simulink model "district_heating_r02"  (R2018b)
settings: Solver=VariableStepAuto  StartTime=0.0  StopTime=24*3600  RelTol=1e-3
undefined symbols (not defined in the file): CollectorBar, DistributorBar, DPConstant, DPLinear, DPQuadratic, FluidMix, ID, MassFlow, path_carnot, Temperature
libraries: carnot x14, Pipe_BiFlow x2
settings Model: Creator=drhf  LastModifiedBy=drhf
settings SolverCC: AlgebraicLoopSolver=LineSearch

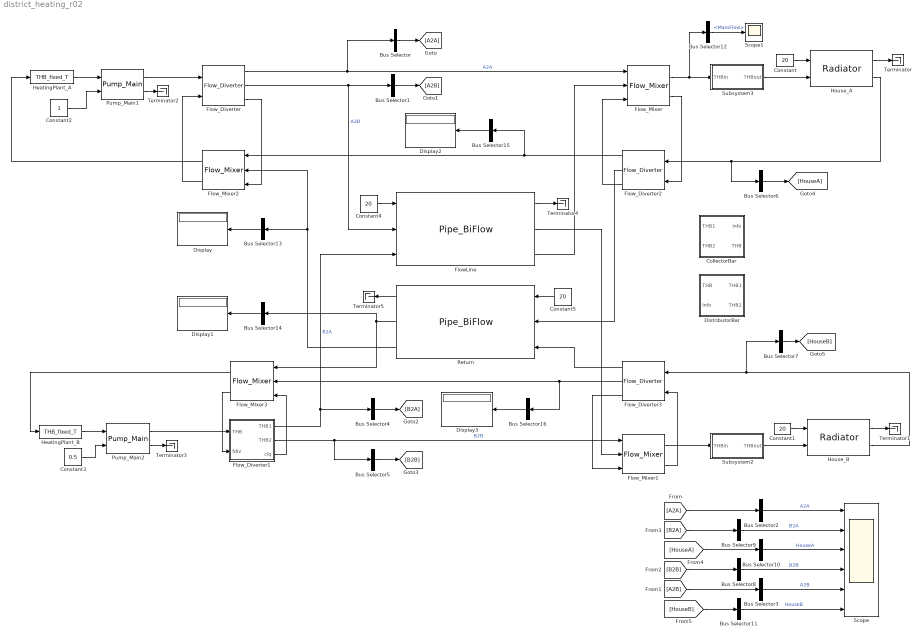
== system district_heating_r02 ==
  Bus Selector{,1,4..7} (6 alike) : BusSelector  OutputSignals=Temperature,MassFlow  OutputAsBus=on
  Bus Selector{2..3,8..11} (6 alike) : BusSelector  OutputSignals=MassFlow  OutputAsBus=on
  Bus Selector12 : BusSelector  OutputSignals=MassFlow
  Bus Selector{13..16} (4 alike) : BusSelector  OutputSignals=DPConstant,DPLinear,DPQuadratic  OutputAsBus=on
  CollectorBar : Subsystem  AncestorBlock=CollectorBar/CollectorBar  mask(Collector bar){}
      mask help: Mixes two massflows. The new temperature is calculated by an energy balance. The "Info" output may be fed back to the corresponding distributor bar.
      mask Help: web(fullfile(path_carnot('help'),'Flow_Mixer.html'),'-helpbrowser')
      mask Display:
      | plot(-50,0, 100,100, ...
      |     [60,60,40,40,60],[10,90,90,10,10], ...
      |     [40,30,30,40],[30,30,20,20], ...
      |     [40,30,30,40],[80,80,70,70], ...
      |     [15,25,15],[30,25,20], ...
      |     [0,25],[25,25], ...
      |     [15,25,15],[80,75,70], ...
      |     [0,25],[75,75])
  Constant{,1,4..5} (4 alike) : Constant  Value=20
  Constant2 : Constant
  Constant3 : Constant  Value=0.5
  Display{,1..3} (4 alike) : Display
  DistributorBar : Subsystem  AncestorBlock=DistributorBar/DistributorBar
      mask Display:
      | plot(0,0,150,100, ...
      |     [60,60,40,40,60],[10,90,90,10,10], ...
      |     [60,70,70,60],[30,30,20,20], ...
      |     [60,70,70,60],[80,80,70,70], ...
      |     [90,100,90],[30,25,20], ...
      |     [75,100],[25,25], ...
      |     [90,100,90],[80,75,70], ...
      |     [75,100],[75,75])
  FlowLine : Pipe_BiFlow/Pipe_BiFlow  t0=20  hgt=254.6479  stgtype=1  tini=[20 20 20 20 20 20 20 20 20 20]  mpts=[1 2 3 4 5 6 7 8 9 10]  PathName=fullfile(path_carnot('libsl'),'Storage','Thermal','Storage_Type_1','parameter_set')  FileName='<user defined>'  userPath=off  userParam=on  uwall=1  ubot=1  utop=1  axcond=1  volume=2  dia=0.1  standing=standing cylinder  nodes=10  mpoints=10  pipe1inlet=1  pipe1outlet=0  pipe1dia=0.1  pipe2inlet=0  pipe2outlet=1  pipe2dia=0.1
  Flow_Diverter : carnot/Hydraulics/Flow_Diverter
      settings: SourceProductName=Carnot
  Flow_Diverter1 : Subsystem  AncestorBlock=carnot/Hydraulics/Flow_Diverter  mask(flow diverter, fixed rate){}
      mask help:
      | The block diverts an incoming massflow according to:
      | mdot1 = mdot * fdiv
      | mdot2 = mdot * (1-fdiv)
      | fdiv is limited to the range [0..1]
      mask Help: web(fullfile(path_carnot('help'),'Flow_Diverter.html'),'-helpbrowser')
      mask Display: plot(0,-5,120,65,[20 45 20 20],[20 30 40 20],[45 70 70 45],[30 20 40 30],[45 35 55 45],[30 10 10 30])
  Flow_Diverter2 : carnot/Hydraulics/Flow_Diverter
      settings: SourceProductName=Carnot
  Flow_Diverter3 : carnot/Hydraulics/Flow_Diverter
      settings: SourceProductName=Carnot
  Flow_Mixer{,1..3} (4 alike) : carnot/Hydraulics/Flow_Mixer
      settings: SourceProductName=Carnot
  HeatingPlant_A : carnot/Source/Simple/THB_fixed_T  t=70
      settings: SourceProductName=Carnot
  HeatingPlant_B : carnot/Source/Simple/THB_fixed_T  t=60
      settings: SourceProductName=Carnot
  House_A : carnot/Source/Heat_Exchanger/Radiator  pnom=500  dtnom=49.83  expo=1.3  mcap=5*4182  tini=20  lin=10  qua=10
      settings: SourceProductName=Carnot
  House_B : carnot/Source/Heat_Exchanger/Radiator  pnom=500  dtnom=49.83  expo=1.3  mcap=5*4182  tini=20  lin=10  qua=10
      settings: SourceProductName=Carnot
  Pump_Main1 : carnot/Hydraulics/Pump_Main  Tini=20  p0=3e5  IDpreset=pressure drop  fluid=Water  mix=0  mix2=0  mix3=0  t1=10  PathName=fullfile(path_carnot('libsl'), 'Hydraulics', 'Pump_Main', 'parameter_set')  FileName='Pump8m.mat'  userPath=off  userParam=off  a0=80000  a1=-32000  a2=0  dia=0.025  UA=1  mcp=4182  e0=100  e1=36  e2=-6.4
      settings: SourceProductName=Carnot
  Pump_Main2 : carnot/Hydraulics/Pump_Main  Tini=20  p0=3e5  IDpreset=pressure drop  fluid=Water  mix=0  mix2=0  mix3=0  t1=10  PathName=fullfile(path_carnot('libsl'), 'Hydraulics', 'Pump_Main', 'parameter_set')  FileName='Pump8m.mat'  userPath=off  userParam=off  a0=80000  a1=-32000  a2=0  dia=0.025  UA=1  mcp=4182  e0=100  e1=36  e2=-6.4
      settings: SourceProductName=Carnot
  Return : Pipe_BiFlow/Pipe_BiFlow  t0=20  hgt=254.6479  stgtype=1  tini=[20 20 20 20 20 20 20 20 20 20]  mpts=[1 2 3 4 5 6 7 8 9 10]  PathName=fullfile(path_carnot('libsl'),'Storage','Thermal','Storage_Type_1','parameter_set')  FileName='<user defined>'  userPath=off  userParam=on  uwall=1  ubot=1  utop=1  axcond=1  volume=2  dia=0.1  standing=standing cylinder  nodes=10  mpoints=10  pipe1inlet=1  pipe1outlet=0  pipe1dia=0.1  pipe2inlet=0  pipe2outlet=1  pipe2dia=0.1
  Scope : Scope  NumInputPorts=6
  Scope1 : Scope
  Subsystem2 : Subsystem
  Subsystem3 : Subsystem
  Terminator{,1..5} (6 alike) : Terminator
  wires:
  Constant/1 -> House_A/1
  House_A/1 -> Terminator/1
  HeatingPlant_B/1 -> Pump_Main2/1
  HeatingPlant_A/1 -> Pump_Main1/1
  House_B/1 -> Terminator1/1
  Constant1/1 -> House_B/1
  Pump_Main1/2 -> Terminator2/1
  Pump_Main2/2 -> Terminator3/1
  Constant2/1 -> Pump_Main1/2
  Constant3/1 -> Pump_Main2/2
  Constant4/1 -> FlowLine/1
  Pump_Main1/1 -> Flow_Diverter/1
  Pump_Main2/1 -> Flow_Diverter1/1(THB)
  FlowLine/1 -> Terminator4/1
  Constant5/1 -> Return/1
  Flow_Diverter/1 -> Flow_Mixer/1, Bus Selector/1  "A2A"
  FlowLine/3 -> Flow_Mixer/2
  Flow_Mixer1/1 -> Subsystem2/1(THBin)
  FlowLine/2 -> Flow_Mixer1/2
  Flow_Diverter1/2(THB2) -> Flow_Mixer1/1, Bus Selector5/1  "B2B"
  House_A/2 -> Bus Selector6/1, Flow_Diverter2/1
  House_B/2 -> Flow_Diverter3/1, Bus Selector7/1
  Return/1 -> Terminator5/1
  Flow_Diverter2/3 -> Flow_Mixer/3
  Flow_Mixer/2 -> Flow_Diverter2/2
  Flow_Mixer1/2 -> Flow_Diverter3/2
  Flow_Diverter3/3 -> Flow_Mixer1/3
  Flow_Diverter1/3(clq) -> Flow_Mixer3/3
  Flow_Mixer3/2 -> Flow_Diverter1/2(fdiv)
  Flow_Mixer2/2 -> Flow_Diverter/2
  Flow_Diverter/3 -> Flow_Mixer2/3
  Flow_Mixer/1 -> Subsystem3/1(THBin), Bus Selector12/1
  Subsystem2/1(THBout) -> House_B/2
  Bus Selector/1 -> [A2A]
  Bus Selector1/1 -> [A2B]
  Flow_Diverter/2 -> FlowLine/2, Bus Selector1/1  "A2B"
  [A2A] -> Bus Selector2/1
  Bus Selector2/1 -> Scope/1  "A2A"
  [A2B] -> Bus Selector3/1
  Bus Selector3/1 -> Scope/5  "A2B"
  Flow_Diverter1/1(THB1) -> FlowLine/3, Bus Selector4/1  "B2A"
  Bus Selector4/1 -> [B2A]
  Bus Selector5/1 -> [B2B]
  Bus Selector6/1 -> [HouseA]
  Bus Selector7/1 -> [HouseB]
  [B2B] -> Bus Selector8/1
  [B2A] -> Bus Selector9/1
  [HouseA] -> Bus Selector10/1
  [HouseB] -> Bus Selector11/1
  Bus Selector8/1 -> Scope/4  "B2B"
  Bus Selector9/1 -> Scope/2  "B2A"
  Bus Selector10/1 -> Scope/3  "HouseA"
  Bus Selector11/1 -> Scope/6  "HouseB"
  Bus Selector12/1 -> Scope1/1  "<MassFlow>"
  Subsystem3/1(THBout) -> House_A/2
  Flow_Mixer2/1 -> HeatingPlant_A/1
  Flow_Mixer3/1 -> HeatingPlant_B/1
  Flow_Diverter2/2 -> Return/2
  Flow_Diverter3/1 -> Return/3
  Return/3 -> Flow_Mixer2/2, Bus Selector13/1
  Return/2 -> Bus Selector14/1, Flow_Mixer3/1
  Bus Selector13/1 -> Display/1
  Bus Selector14/1 -> Display1/1
  Flow_Diverter2/1 -> Bus Selector15/1, Flow_Mixer2/1
  Bus Selector15/1 -> Display2/1
  Flow_Diverter3/2 -> Bus Selector16/1, Flow_Mixer3/2
  Bus Selector16/1 -> Display3/1

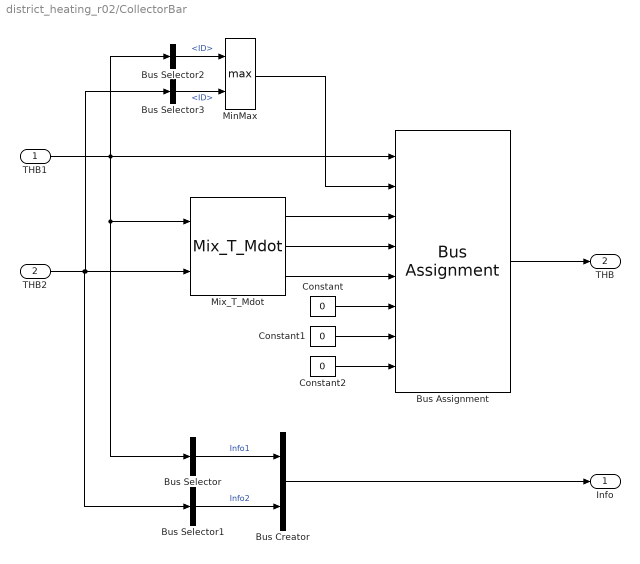
== system district_heating_r02/CollectorBar ==
  THB1 : Inport
  THB2 : Inport  Port=2
  Bus Assignment : BusAssignment  AssignedSignals=ID,Temperature,MassFlow,FluidMix,DPConstant,DPLinear,DPQuadratic
  Bus Creator : BusCreator  Inputs=2
  Bus Selector : BusSelector  OutputSignals=MassFlow,DPConstant,DPLinear,DPQuadratic  OutputAsBus=on
  Bus Selector1 : BusSelector  OutputSignals=MassFlow,DPConstant,DPLinear,DPQuadratic  OutputAsBus=on
  Bus Selector2 : BusSelector  OutputSignals=ID
  Bus Selector3 : BusSelector  OutputSignals=ID
  Constant : Constant  Value=0
  Constant1 : Constant  Value=0
  Constant2 : Constant  Value=0
  MinMax : MinMax  Function=max  Inputs=2
  Mix_T_Mdot : carnot/Basic/Hydraulics/Mix_T_Mdot  mixcalc=Tmix = (mdot1*T1 + mdot2*T2)/(mdot1+mdot2)
      settings: SourceProductName=Carnot
  Info : Outport
  THB : Outport  Port=2
  wires:
  Bus Creator/1 -> Info/1
  Bus Selector1/1 -> Bus Creator/2  "Info2"
  Bus Selector/1 -> Bus Creator/1  "Info1"
  Constant2/1 -> Bus Assignment/8
  Constant1/1 -> Bus Assignment/7
  Constant/1 -> Bus Assignment/6
  Mix_T_Mdot/3 -> Bus Assignment/5
  Mix_T_Mdot/2 -> Bus Assignment/4
  Mix_T_Mdot/1 -> Bus Assignment/3
  Bus Assignment/1 -> THB/1
  THB2/1 -> Bus Selector1/1, Bus Selector3/1, Mix_T_Mdot/2
  THB1/1 -> Bus Selector/1, Mix_T_Mdot/1, Bus Selector2/1, Bus Assignment/1
  Bus Selector2/1 -> MinMax/1  "<ID>"
  Bus Selector3/1 -> MinMax/2  "<ID>"
  MinMax/1 -> Bus Assignment/2

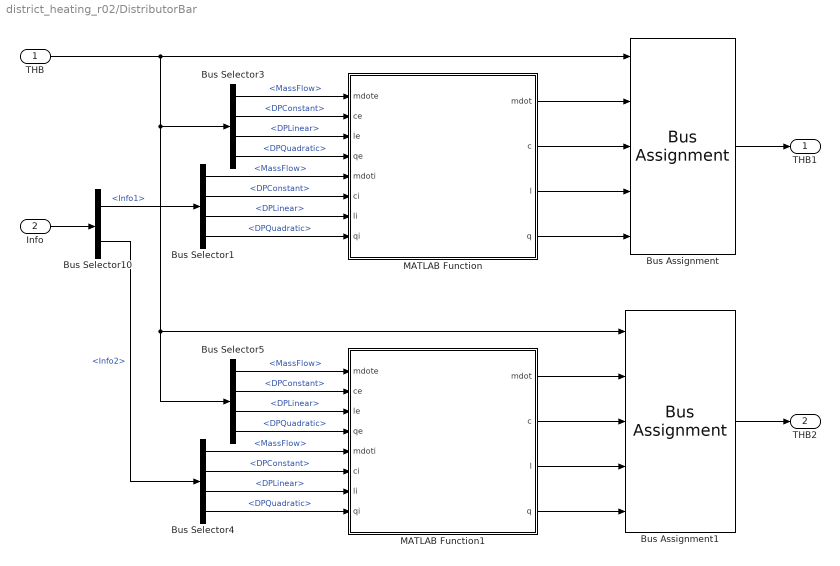
== system district_heating_r02/DistributorBar ==
  THB : Inport
  Info : Inport  Port=2
  Bus Assignment : BusAssignment  AssignedSignals=MassFlow,DPConstant,DPLinear,DPQuadratic
  Bus Assignment1 : BusAssignment  AssignedSignals=MassFlow,DPConstant,DPLinear,DPQuadratic
  Bus Selector{1,3..5} (4 alike) : BusSelector  OutputSignals=MassFlow,DPConstant,DPLinear,DPQuadratic
  Bus Selector10 : BusSelector  OutputSignals=Info1,Info2
  MATLAB Function : MATLAB Function  TreatAsAtomicUnit=on
  MATLAB Function1 : MATLAB Function  TreatAsAtomicUnit=on
  THB1 : Outport
  THB2 : Outport  Port=2
  wires:
  Bus Selector10/2 -> Bus Selector4/1  "<Info2>"
  MATLAB Function1/3(l) -> Bus Assignment1/4
  MATLAB Function1/4(q) -> Bus Assignment1/5
  MATLAB Function1/1(mdot) -> Bus Assignment1/2
  MATLAB Function1/2(c) -> Bus Assignment1/3
  Bus Selector4/4 -> MATLAB Function1/8(qi)  "<DPQuadratic>"
  Bus Selector4/3 -> MATLAB Function1/7(li)  "<DPLinear>"
  Bus Selector4/2 -> MATLAB Function1/6(ci)  "<DPConstant>"
  Bus Selector4/1 -> MATLAB Function1/5(mdoti)  "<MassFlow>"
  Bus Selector5/1 -> MATLAB Function1/1(mdote)  "<MassFlow>"
  Bus Selector5/2 -> MATLAB Function1/2(ce)  "<DPConstant>"
  Bus Selector5/3 -> MATLAB Function1/3(le)  "<DPLinear>"
  Bus Selector5/4 -> MATLAB Function1/4(qe)  "<DPQuadratic>"
  Bus Selector1/4 -> MATLAB Function/8(qi)  "<DPQuadratic>"
  Bus Selector1/3 -> MATLAB Function/7(li)  "<DPLinear>"
  Bus Selector1/2 -> MATLAB Function/6(ci)  "<DPConstant>"
  Bus Selector1/1 -> MATLAB Function/5(mdoti)  "<MassFlow>"
  Bus Selector3/1 -> MATLAB Function/1(mdote)  "<MassFlow>"
  Bus Selector3/2 -> MATLAB Function/2(ce)  "<DPConstant>"
  Bus Selector3/3 -> MATLAB Function/3(le)  "<DPLinear>"
  Bus Selector3/4 -> MATLAB Function/4(qe)  "<DPQuadratic>"
  MATLAB Function/4(q) -> Bus Assignment/5
  MATLAB Function/3(l) -> Bus Assignment/4
  MATLAB Function/2(c) -> Bus Assignment/3
  MATLAB Function/1(mdot) -> Bus Assignment/2
  Bus Selector10/1 -> Bus Selector1/1  "<Info1>"
  Bus Assignment1/1 -> THB2/1
  Bus Assignment/1 -> THB1/1
  THB/1 -> Bus Assignment1/1, Bus Selector5/1, Bus Selector3/1, Bus Assignment/1
  Info/1 -> Bus Selector10/1

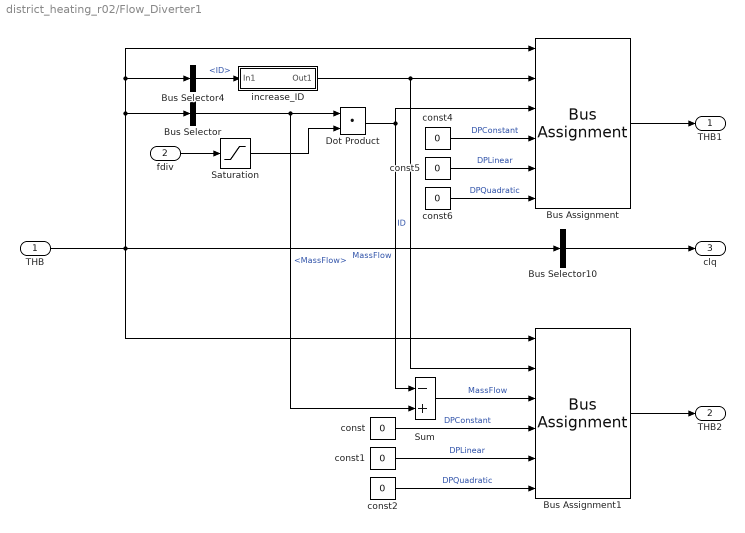
== system district_heating_r02/Flow_Diverter1 ==
  THB : Inport
  fdiv : Inport  Port=2
  Bus Assignment : BusAssignment  AssignedSignals=ID,MassFlow,DPConstant,DPLinear,DPQuadratic
  Bus Assignment1 : BusAssignment  AssignedSignals=ID,MassFlow,DPConstant,DPLinear,DPQuadratic
  Bus Selector10 : BusSelector  OutputSignals=MassFlow,DPConstant,DPLinear,DPQuadratic  OutputAsBus=on
  Bus Selector : BusSelector  OutputSignals=MassFlow
  Bus Selector4 : BusSelector  OutputSignals=ID
  Dot Product : DotProduct  InputSameDT=on  OutDataTypeStr=Inherit: Inherit via internal rule
  Saturation : Saturate  UpperLimit=1  LowerLimit=0
  Sum : Sum  Inputs=-+  SaturateOnIntegerOverflow=on  InputSameDT=on  OutDataTypeStr=Inherit: Same as first input
  const{,1..2,4..6} (6 alike) : Constant  Value=0
  increase_ID : Subsystem
  THB1 : Outport
  THB2 : Outport  Port=2
  clq : Outport  Port=3
  wires:
  const2/1 -> Bus Assignment1/6  "DPQuadratic"
  const1/1 -> Bus Assignment1/5  "DPLinear"
  Saturation/1 -> Dot Product/2
  Sum/1 -> Bus Assignment1/3  "MassFlow"
  Bus Selector/1 -> Dot Product/1, Sum/2  "<MassFlow>"
  const/1 -> Bus Assignment1/4  "DPConstant"
  THB/1 -> Bus Selector/1, Bus Assignment/1, Bus Selector4/1, Bus Selector10/1, Bus Assignment1/1
  fdiv/1 -> Saturation/1
  Dot Product/1 -> Sum/1, Bus Assignment/3  "MassFlow"
  Bus Selector4/1 -> increase_ID/1(In1)  "<ID>"
  increase_ID/1(Out1) -> Bus Assignment/2, Bus Assignment1/2  "ID"
  const6/1 -> Bus Assignment/6  "DPQuadratic"
  const5/1 -> Bus Assignment/5  "DPLinear"
  const4/1 -> Bus Assignment/4  "DPConstant"
  Bus Assignment/1 -> THB1/1
  Bus Assignment1/1 -> THB2/1
  Bus Selector10/1 -> clq/1

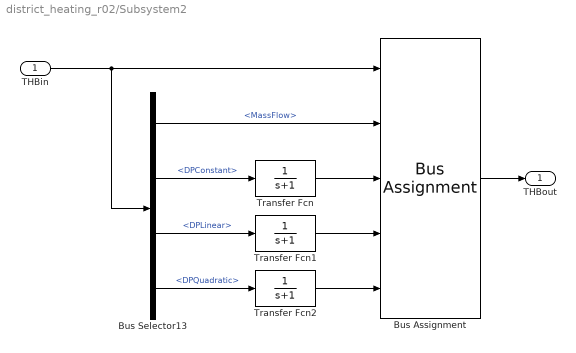
== system district_heating_r02/Subsystem2 ==
  THBin : Inport
  Bus Assignment : BusAssignment  AssignedSignals=MassFlow,DPConstant,DPLinear,DPQuadratic
  Bus Selector13 : BusSelector  OutputSignals=MassFlow,DPConstant,DPLinear,DPQuadratic
  Transfer Fcn : TransferFcn  Denominator=[1 1]
  Transfer Fcn1 : TransferFcn  Denominator=[1 1]
  Transfer Fcn2 : TransferFcn  Denominator=[1 1]
  THBout : Outport
  wires:
  Transfer Fcn2/1 -> Bus Assignment/5
  Transfer Fcn1/1 -> Bus Assignment/4
  Transfer Fcn/1 -> Bus Assignment/3
  Bus Selector13/4 -> Transfer Fcn2/1  "<DPQuadratic>"
  Bus Selector13/3 -> Transfer Fcn1/1  "<DPLinear>"
  Bus Selector13/2 -> Transfer Fcn/1  "<DPConstant>"
  Bus Selector13/1 -> Bus Assignment/2  "<MassFlow>"
  THBin/1 -> Bus Selector13/1, Bus Assignment/1
  Bus Assignment/1 -> THBout/1

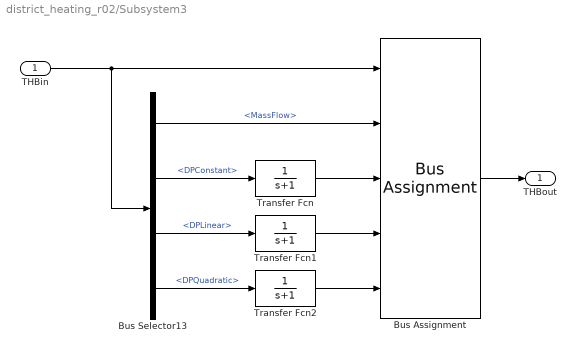
== system district_heating_r02/Subsystem3 ==
  THBin : Inport
  Bus Assignment : BusAssignment  AssignedSignals=MassFlow,DPConstant,DPLinear,DPQuadratic
  Bus Selector13 : BusSelector  OutputSignals=MassFlow,DPConstant,DPLinear,DPQuadratic
  Transfer Fcn : TransferFcn  Denominator=[1 1]
  Transfer Fcn1 : TransferFcn  Denominator=[1 1]
  Transfer Fcn2 : TransferFcn  Denominator=[1 1]
  THBout : Outport
  wires:
  Bus Assignment/1 -> THBout/1
  THBin/1 -> Bus Assignment/1, Bus Selector13/1
  Bus Selector13/1 -> Bus Assignment/2  "<MassFlow>"
  Bus Selector13/2 -> Transfer Fcn/1  "<DPConstant>"
  Bus Selector13/3 -> Transfer Fcn1/1  "<DPLinear>"
  Bus Selector13/4 -> Transfer Fcn2/1  "<DPQuadratic>"
  Transfer Fcn/1 -> Bus Assignment/3
  Transfer Fcn1/1 -> Bus Assignment/4
  Transfer Fcn2/1 -> Bus Assignment/5

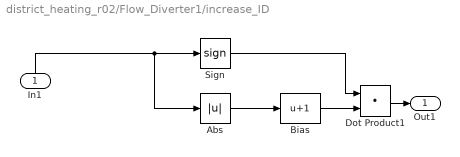
== system district_heating_r02/Flow_Diverter1/increase_ID ==
  In1 : Inport
  Abs : Abs
  Bias : Bias  Bias=1
  Dot Product1 : DotProduct  InputSameDT=on  OutDataTypeStr=Inherit: Inherit via internal rule
  Sign : Signum
  Out1 : Outport
  wires:
  Bias/1 -> Dot Product1/2
  Sign/1 -> Dot Product1/1
  Abs/1 -> Bias/1
  Dot Product1/1 -> Out1/1
  In1/1 -> Sign/1, Abs/1

== matlab function district_heating_r02/DistributorBar/MATLAB Function1 ==
  data: mdot output; mdote input; c output; ce input; le input; qe input; l output; q output; mdoti input; ci input; li input; qi input
function [mdot, c, l, q] = distributorBar_recalc_clq(mdote, ce, le, qe, mdoti, ci, li, qi)

% Basic equations:
% pressure drop dp = c + l*mdot + q*mdot^2

noMassflow = sqrt(eps(100));  % assume no massflow below this limit

% Massflow mdoti in the branch is given via info inport .
mdot = mdoti; % massflow is flow from info input

% Entering flow mdote and its coeffs (ce, le, qe) must be replaced by
% mdoti  with coeffs c, l, q fullfilling the condition that
% calulated pressure drop in entering pipe is maintained
%  dp = ce + le*mdote + qe*mdote^2 =  c + l*mdoti + q*mdoti^2 
% for all massflows mdote and mdoti
% -> c = ce
% -> l = le*mdote/mdoti
% -> q = qe*mdote^2/mdoti^2
c = ce;
if mdoti < noMassflow
    l = le;
    q = qe;
else
    v = mdote/mdoti;
    l = le*v;
    q = qe*v^2;
end

% additional pressure drop from the info inport must be added
c = c + ci;
l = l + li;
q = q + qi;

== matlab function district_heating_r02/DistributorBar/MATLAB Function ==
  data: mdot output; mdote input; c output; ce input; le input; qe input; l output; q output; mdoti input; ci input; li input; qi input
function [mdot, c, l, q] = distributorBar_recalc_clq(mdote, ce, le, qe, mdoti, ci, li, qi)

% Basic equations:
% pressure drop dp = c + l*mdot + q*mdot^2

noMassflow = sqrt(eps(100));  % assume no massflow below this limit

% Massflow mdoti in the branch is given via info inport .
mdot = mdoti; % massflow is flow from info input

% Entering flow mdote and its coeffs (ce, le, qe) must be replaced by
% mdoti  with coeffs c, l, q fullfilling the condition that
% calulated pressure drop in entering pipe is maintained
%  dp = ce + le*mdote + qe*mdote^2 =  c + l*mdoti + q*mdoti^2 
% for all massflows mdote and mdoti
% -> c = ce
% -> l = le*mdote/mdoti
% -> q = qe*mdote^2/mdoti^2
c = ce;
if mdoti < noMassflow
    l = le;
    q = qe;
else
    v = mdote/mdoti;
    l = le*v;
    q = qe*v^2;
end

% additional pressure drop from the info inport must be added
c = c + ci;
l = l + li;
q = q + qi;
